simulink model "stm32f0_ccp_sensor"  (Simulink 7.3)
settings: Solver=ode3  SolverMode=SingleTasking  StartTime=0.0  StopTime=10.0  RelTol=1e-3
PreLoadFcn:
  | waijung.modelPreload; % Required for working with Waijung Blockset. Do not remove.
undefined symbols (not defined in the file): ARM, LQFP48, MDK, STM32F072CB
libraries: simulink x216, waijung_soft_i2c_lib x28, waijung_addon_module x12, stm32f0_flash_lib x10, stm32f0_can_lib x3, stm32f0_reset_lib x1, waijung_crc_lib x1, stm32f0_boot_lib x1, stm32f0_device_config_lib x1
(part 1 of 6)
CloseFcn:
  | waijung.modelClose; % Required for working with Waijung Blockset. Do not remove.
settings Model: Creator=Nav  LastModifiedBy=Krisada
settings OptimizationCC: OptimizeModelRefInitCode=on  LifeSpan=1
settings HardwareCC: ProdEndianess=LittleEndian  ProdHWDeviceType=ARM Compatible->Cortex - M0  TargetEndianess=LittleEndian  TargetHWDeviceType=ARM Compatible->Cortex - M0
settings RTWCC: SystemTargetFile=stm32f0.tlc  GenerateMakefile=off  TemplateMakefile=ert_default_tmf  Description=STM32F0 Target  ProcessScript=stm32f0_make_rtw_hook
settings CodeAppCC: IgnoreCustomStorageClasses=off
settings STFCustomTargetCC: ModelReferenceCompliant=off  CombineOutputUpdateFcns=on  ERTCustomFileBanners=on  SupportNonInlinedSFcns=off  SystemTargetFile=stm32f0.tlc
settings ERTTargetCC: MultiwordLength=2048  ModelReferenceCompliant=off  ParMdlRefBuildCompliant=off  CompOptLevelCompliant=off  ERTFirstTimeCompliant=off  SupportContinuousTime=on  ModelStepFunctionPrototypeControlCompliant=off  CPPClassGenCompliant=off  ExtModeMexFile=noextcomm  InlinedParameterPlacement=NonHierarchical  ERTSrcFileBannerTemplate=stm32f0_code_template.cgt  ERTHdrFileBannerTemplate=stm32f0_code_template.cgt  ERTDataSrcFileTemplate=stm32f0_code_template.cgt  ERTDataHdrFileTemplate=stm32f0_code_template.cgt  ERTCustomFileTemplate=stm32f0_file_process.tlc

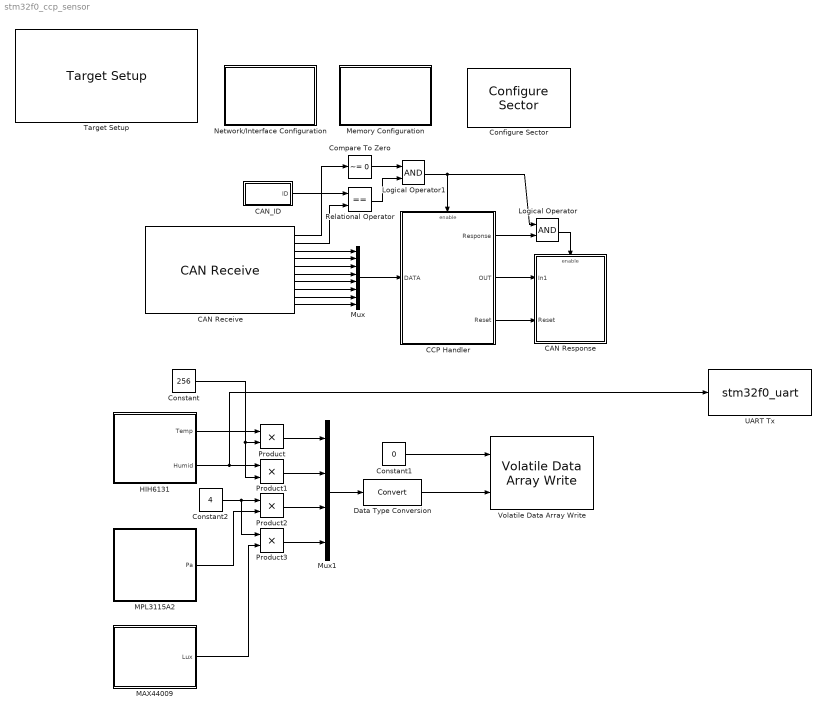
== system stm32f0_ccp_sensor ==
  CAN Receive : stm32f0_can_lib/CAN Receive  conf=Rx  canmodule=1  idtype=Standard  filtertype=Mask  id=0  idmask=0  enableisr=off  usedlc=off  datatype=single  data0type=uint8  data1type=uint8  data2type=uint8  data3type=uint8  data4type=uint8  data5type=uint8  data6type=uint8  data7type=uint8  buffersize=8  sampletime=0.01  sampletimestr=0.01  blockid=CANReceive  inputarray=[]  inputlabelarray={}  outputarray=[ 5, 7, 3, 3, 3, 3, 3, 3, 3, 3]  outputlabelarray={ 'Msg Pending','ID', 'D0 (uint8)', 'D1 (uint8)', 'D2 (uint8)', 'D3 (uint8)', 'D4 (uint8)', 'D5 (uint8)', 'D6 (uint8)', 'D7 (uint8)' }  compat=0  confstr="[\"Standard\",\"Mask\",\"0\",\"0\",\"off\",\"uint8\",\"uint8\",\"uint8\",\"uint8\",\"uint8\",\"uint8\",\"uint8\",\"uint8\",\"8\",\"0\",\"0\",\"0\",\"4\"]"
  CAN Response : Subsystem
  CAN_ID : Subsystem
  CCP Handler : Subsystem  TreatAsAtomicUnit=on
  Compare To Zero : simulink/Logic and Bit Operations/Compare To Zero  SystemSampleTime=-1  relop=~=  LogicOutDataTypeMode=uint8  ZeroCross=off
  Configure Sector : stm32f0_boot_lib/Configure Sector  conf=Configure  flashorigin=0x8004000  flashlength=0x00D000  enableisr=off  usersector=Sector 5: 0x08020000 - 0x0803FFFF  sampletime=-1  sampletimestr=0.01  blockid=ConfigureSector  inputarray=[]  inputlabelarray={}  outputarray=[]  outputlabelarray={}  compat=0  confstr="[\"8020000\",\"5\",\"8004000\"]"
  Constant : Constant  Value=256  OutDataTypeMode=uint32  OutDataType=fixdt(1, 16)  OutScaling=2^0  OutDataTypeStr=uint32
  Constant1 : Constant  Value=0  OutDataTypeMode=uint32  OutDataType=fixdt(1, 16)  OutScaling=2^0  OutDataTypeStr=uint32
  Constant2 : Constant  Value=4  OutDataTypeMode=uint32  OutDataType=fixdt(1, 16)  OutScaling=2^0  OutDataTypeStr=uint32
  Data Type Conversion : DataTypeConversion  OutDataType=fixdt(1, 16)  OutScaling=2^0
  HIH6131 : Subsystem
  Logical Operator : Logic  AllPortsSameDT=off  OutDataTypeMode=boolean  LogicDataType=fixdt(0, 8)  OutDataTypeStr=boolean
  Logical Operator1 : Logic  AllPortsSameDT=off  OutDataTypeMode=boolean  LogicDataType=fixdt(0, 8)  OutDataTypeStr=boolean
  MAX44009 : Subsystem
  MPL3115A2 : Subsystem
  Memory Configuration : Subsystem
  Mux : Mux  Inputs=8
  Mux1 : Mux
  Network/Interface Configuration : Subsystem
  Product{,1..3} (4 alike) : Product  OutDataType=fixdt(1, 16)  OutScaling=2^0  RndMeth=Zero
  Relational Operator : RelationalOperator  Operator===  LogicOutDataTypeMode=boolean  LogicDataType=fixdt(0, 8)  OutDataTypeStr=boolean
  Target Setup : stm32f0_device_config_lib/Target Setup  Priority=100  compiler=MDK-ARM  previous_compiler=MDK-ARM  mcu=STM32F072CB (LQFP48)  mcustr=STM32F072CB  stdlib=STM32F072  clockconfig=STM32F072B-DISCO Default (HSIOSC-8MHz/HCLK-48MHz)  system_stm32f0xx_c_path=F:\trunk\targets\stm32f0_target\stm32f0\utils\STM32F0xx_AN4055\stm32f0_default\hsi8mhz_pll_hclk48mhz  showmemoryconfiguration=on  stacksize=0x400  heapsize=0x200  enableautocompiledownload=on  fullchiperase=off  programmerinterface=None  editctrlstr=on  compilercontrolstr=-c --cpu Cortex-M0 -O3 --apcs=interwork --split_sections $(INCLUDES)  assemblercontrolstr=--cpu Cortex-M0 --apcs=interwork --xref $(INCLUDES)  linkercontrolstr="--cpu Cortex-M0 --strict --scatter \"$(MODELNAME).sct\" --summary_stderr --info summarysizes --map --xref --callgraph --symbols --info sizes --info totals --info unused --info veneers  --list \".\\$(MODELNAME).map\" -o $(MODELNAME).axf"  runafterdownload=on  execprofile=None  profileruart=3  profilerbaud=500000  profilertxpin=Not used  profilerinitstr=0.01,48000000,480000,500000,0  manualsetsampletime=on  sampletime=0.01  blockid=TargetSetup  systickreloadvalue=480000  hseval=8000000  lastprofileruart=3  hclk=48000000  flashorigin=0x8004000  flashlength=0x00D000  ramorigin=0x20000000  ramlength=0x00004000  useextram=off
  UART Tx : S-Function  FunctionName=stm32f0_uart  Parameters=conf,inputporttype,inputportwidth,outputporttype,outputportwidth,asciiheader,optionstring,headerstring,terminatorstring,asciidatatypestring,sampletime,blockid  EnableBusSupport=off  mask(stm32f0_uart){conf=Tx, uartmodule=1, baudrate=115200, databits=8, parity=No, stopbit=1, remaptxpin=A9, remaprxpin=A10, flowcontrol=None, remapctspin=Not used, remaprtspin=Not used, advanceoptions=off, rxbuffersize=64, txbuffersize=64, transfer=Non-Blocking, packetmode=Ascii, binheader='7E 7E', binterminator='03 03', porttype_double=0, porttype_single=0, porttype_int8=0, porttype_uint8=0, porttype_int16=0, porttype_uint16=0, porttype_int32=0, porttype_uint32=2, asciiformat='%1.2f', rx_asciiterminator=CR (0x0D - "\r"), tx_asciiterminator=CRLF (0x0D 0x0A - "\r\n"), storagename=<empty>, varname=, asciiheader=%1.2f\r\n, sampletime=inf, enablecustomportlabel=off, cinputportlabel=de, coutputportlabel=fff,ff,sdfsd, portpinstr=0, blockid=UARTTx, inputporttype=[ -1], inputportwidth=[], inputportlabel={ '%f'}, outputporttype=[], outputportwidth=[], outputportlabel={}, compat=0, optionstring=["1", "1", "A", "9", "1", "A", "10", "0", "*", "*", "0", "*", "*", "1", "1", "", "", "115200", "8", "No", "1", "None", "3", "2", "64", "64", "Ascii", "Non-Blocking", ""], headerstring=[], terminatorstring=["13","10"], asciidatatypestring=["float"], lastmodule=1}
      mask prompts: conf "Configuration"; uartmodule "UART Module"; baudrate "Baud rate (bps)"; databits "Data bits"; stopbit "Stop bit"; remaptxpin "Tx pin"; remaprxpin "Rx pin"; flowcontrol "Hardware flow control"; remapctspin "HW Flow control, CTS Pin"; remaprtspin "HW Flow control, RTS Pin"; advanceoptions "Advance options"; rxbuffersize "Rx buffer size (bytes)"; txbuffersize "Tx buffer size (bytes)"; packetmode "Packet mode"; binheader "Binary header (example: '7E 7E')"; binterminator "Binary terminator (example: '03 03')"; porttype_double "Number of data port, type DOUBLE"; porttype_single "Number of data port, type SINGLE"; porttype_int8 "Number of data port, type INT8"; porttype_uint8 "Number of data port, type UINT8"; porttype_int16 "Number of data port, type INT16"; porttype_uint16 "Number of data port, type UINT16"; porttype_int32 "Number of data port, type INT32"; porttype_uint32 "Number of data port, type UINT32"; asciiformat "Ascii format"; rx_asciiterminator "End of packet"; tx_asciiterminator "End of packet"; storagename "Buffer"; varname "Var name"; asciiheader "Ascii header (printf format)"; sampletime "Sample time (sec)"; enablecustomportlabel "Enable custom port labels (Ex. In1, In2, In3)"; cinputportlabel "Custom input port labels (Ex. In1, In2, In3)"; coutputportlabel "Custom output port labels (Ex. Out1, Out2, Out3)"; portpinstr "Port Pin String"; blockid "Block ID"; inputporttype "Input Port Type"; inputportwidth "Input Port Width"; inputportlabel "Input Port Label"; outputporttype "Output Port Type"; outputportwidth "Output Port Width"; outputportlabel "Output port label"; compat "Compatibility (Reserved for future use)"; optionstring "String(s) to be passed to TLC"; lastmodule "Last module selected"
      mask help:
      | UART Module
      |  - Select module corresponding to "UART Setup" block.
      | Transfer
      |  - Blocking: after write DMA buffer, the block wait until buffer empty.
      |  - Non-Blocking: the block will not wait for buffer empty.
      | Packet mode:
      |  - Ascii: sending data is ascii, Ascii format + End of packet.
      |  - Binary: sending data is binary format, Header + Data + Terminator
      |  - String Buffer: Volatile Data Storage variable name as sending data.
      | Ascii format:
      |  - %U, %I, %D, %O, %X, %u, %i, %d, %o, %x: Uint32
      |  - %E, %G, %F, %e, %g, %f: Single
      |  - %C, %c: Int8
      |  - %S, %s: (char *), this port is output of Volatile Data Storage Read block, which data type is string.
      mask init:
      | stm32f0_uart_callback('init');
      mask Help: web(fullfile(waijungdocroot,'stm32f0_uart_tx.htm'), '-browser')
      mask StyleString: popup(Setup|Tx|Rx),popup(1|2|3|4),edit,popup(8),popup(No|Odd|Even),popup(0.5|1|1.5|2),popup(Not used|A9|B6),popup(Not used|A10|B7),popup(None|RTS|CTS|RTS/CTS),popup(Not used|A11),popup(Not used|A12),checkbox,popup(16|32|64|128|256|512),popup(16|32|64|128|256|512),popup(Blocking|Non-Blocking),popup(Ascii|Binary|String Buffer),edit,edit,edit,edit,edit,edit,edit,edit,edit,edit,edit,popup(CR (0x0D - "\r")|LF (0x0A - "\n")|CRLF (0x0D 0x0A - "\r\n")),popup(CR (0x0D - "\r")|LF (0x0A - "\n")|CRLF (0x0D 0x0A - "\r\n")|None),popup(<empty>),edit,edit,edit,checkbox,edit,edit,edit,edit,edit,edit,edit,edit,edit,edit,edit,edit,edit,edit,edit,edit
      mask CallbackString: stm32f0_uart_callback('conf');|stm32f0_uart_callback('uartmodule');|||||||stm32f0_uart_callback('flowcontrol');|||stm32f0_uart_callback('advanceoptions');|||stm32f0_uart_callback('conf');|stm32f0_uart_callback('conf');|stm32f0_uart_callback('binheader');|stm32f0_uart_callback('binterminator');|||||||||stm32f0_uart_callback('asciiformat');|||stm32f0_uart_callback('storagename');|||stm32f0_uart_callback('sampletime');|stm32f0_uart_callback('enablecustomportlabel');|stm32f0_uart_callback('conf');|stm32f0_uart_callback('conf');||stm32f0_uart_callback('blockid');||||||||||||
      mask Display: text(0.95, 0.5, 'Module: USART1_Tx\nPacket: Ascii\nTransfer: Non-Blocking\nTs (sec): 0.5','ver','middle','hor','right'); port_label('input', 1,'%f');
  Volatile Data Array Write : waijung_addon_module/Data Storage/Volatile Data Array Write  conf=Write  specificaddress=off  storagename=READ_DATA  memoryaddress=hex2dec('64000000')  storagetype=uint8  datasize=120*160*3  varname=VolatileDataArray_READ_DATA  datatype=uint32  datacount=4  variablesize=off  portpinstr=0  sampletime=inf  blockid=VolatileDataArrayWrite  inputporttype=[7 7]  inputportwidth=[1 4]  inputportlabel={'Offset', 'Data'}  outputporttype=[]  outputportwidth=[]  outputportlabel={}  compat=0  optionstring="[\"READ_DATA\",\"uint8\",\"256\",\"VolatileDataArray_READ_DATA\",\"uint8_t\",\"uint32\",\"uint32_t\",\"4\",\"Param1\"]"
  wires:
  CAN Receive/1 -> Compare To Zero/1
  CAN Receive/3 -> Mux/1
  CAN Receive/4 -> Mux/2
  CAN Receive/5 -> Mux/3
  CAN Receive/6 -> Mux/4
  CAN Receive/7 -> Mux/5
  CAN Receive/8 -> Mux/6
  CAN Receive/9 -> Mux/7
  CAN Receive/10 -> Mux/8
  Mux/1 -> CCP Handler/1(DATA)
  CAN Receive/2 -> Relational Operator/2
  CCP Handler/2(OUT) -> CAN Response/1(In1)
  CCP Handler/1(Response) -> Logical Operator/2
  Logical Operator/1 -> CAN Response/Enable
  CCP Handler/3(Reset) -> CAN Response/2(Reset)
  CAN_ID/1(ID) -> Relational Operator/1
  Compare To Zero/1 -> Logical Operator1/1
  Logical Operator1/1 -> CCP Handler/Enable, Logical Operator/1
  Mux1/1 -> Data Type Conversion/1
  Product/1 -> Mux1/1
  Product1/1 -> Mux1/2
  Constant/1 -> Product/2, Product1/2
  Relational Operator/1 -> Logical Operator1/2
  HIH6131/1(Temp) -> Product/1
  HIH6131/2(Humid) -> Product1/1, UART Tx/1
  Product2/1 -> Mux1/3
  Constant2/1 -> Product2/1, Product3/1
  MPL3115A2/1(Pa) -> Product2/2
  Product3/1 -> Mux1/4
  MAX44009/1(Lux) -> Product3/2
  Constant1/1 -> Volatile Data Array Write/1
  Data Type Conversion/1 -> Volatile Data Array Write/2

== system stm32f0_ccp_sensor/CAN Response ==
  In1 : Inport
  Reset : Inport  Port=2
  Enable : EnablePort
  CAN Transmit : stm32f0_can_lib/CAN Transmit  conf=Tx  canmodule=1  transfer=Blocking  timeout=0.1  idtype=Standard  specificid=on  id=255  specificdlc=on  dlc=8  enablestatus=on  datatype=single  data0type=uint8  data1type=uint8  data2type=uint8  data3type=uint8  data4type=uint8  data5type=uint8  data6type=uint8  data7type=uint8  inputarray=[ 3, 3, 3, 3, 3, 3, 3, 3]  inputlabelarray={ 'D0 (uint8)', 'D1 (uint8)', 'D2 (uint8)', 'D3 (uint8)', 'D4 (uint8)', 'D5 (uint8)', 'D6 (uint8)', 'D7 (uint8)' }  outputarray=[7]  outputlabelarray={'Status'}  sampletime=-1  sampletimestr=0.01  blockid=CANResponseCANTransmit  compat=0  confstr="[\"Blocking\",\"0.1\",\"Standard\",\"on\",\"255\",\"on\",\"8\",\"on\",\"uint8\",\"uint8\",\"uint8\",\"uint8\",\"uint8\",\"uint8\",\"uint8\",\"uint8\"]"
  Compare To Zero : simulink/Logic and Bit Operations/Compare To Zero  SystemSampleTime=-1  relop===  LogicOutDataTypeMode=boolean  ZeroCross=off
  Demux : Demux  Outputs=8
  Demux1 : Demux  Outputs=8
  Logical Operator : Logic  AllPortsSameDT=off  OutDataTypeMode=boolean  LogicDataType=fixdt(0, 8)  OutDataTypeStr=boolean
  Reboot : Subsystem  TreatAsAtomicUnit=on
  UART Tx : S-Function  FunctionName=stm32f0_uart  Parameters=conf,inputporttype,inputportwidth,outputporttype,outputportwidth,asciiheader,optionstring,headerstring,terminatorstring,asciidatatypestring,sampletime,blockid  EnableBusSupport=off  mask(stm32f0_uart){conf=Tx, uartmodule=1, baudrate=115200, databits=8, parity=No, stopbit=1, remaptxpin=A9, remaprxpin=A10, flowcontrol=None, remapctspin=Not used, remaprtspin=Not used, advanceoptions=off, rxbuffersize=64, txbuffersize=64, transfer=Non-Blocking, packetmode=Ascii, binheader='7E 7E', binterminator='03 03', porttype_double=0, porttype_single=0, porttype_int8=0, porttype_uint8=0, porttype_int16=0, porttype_uint16=0, porttype_int32=0, porttype_uint32=2, asciiformat='TX: %X,%X,%X,%X,%X,%X,%X,%X: %u', rx_asciiterminator=CR (0x0D - "\r"), tx_asciiterminator=CRLF (0x0D 0x0A - "\r\n"), storagename=<empty>, varname=, asciiheader=TX: %X,%X,%X,%X,%X,%X,%X,%X: %u\r\n, sampletime=inf, enablecustomportlabel=off, cinputportlabel=de, coutputportlabel=fff,ff,sdfsd, portpinstr=0, blockid=CANResponseUARTTx, inputporttype=[ -1 -1 -1 -1 -1 -1 -1 -1 -1], inputportwidth=[], inputportlabel={ '%X' '%X' '%X' '%X' '%X' '%X' '%X' '%X' '%u'}, outputporttype=[], outputportwidth=[], outputportlabel={}, compat=0, optionstring=["1", "1", "A", "9", "1", "A", "10", "0", "*", "*", "0", "*", "*", "1", "1", "", "", "115200", "8", "No", "1", "None", "3", "2", "64", "64", "Ascii", "Non-Blocking", ""], headerstring=[], terminatorstring=["13","10"], asciidatatypestring=["uint32_t","uint32_t","uint32_t","uint32_t","uint32_t","uint32_t","uint32_t","uint32_t","uint32_t"], lastmodule=1}
      mask prompts: conf "Configuration"; uartmodule "UART Module"; baudrate "Baud rate (bps)"; databits "Data bits"; stopbit "Stop bit"; remaptxpin "Tx pin"; remaprxpin "Rx pin"; flowcontrol "Hardware flow control"; remapctspin "HW Flow control, CTS Pin"; remaprtspin "HW Flow control, RTS Pin"; advanceoptions "Advance options"; rxbuffersize "Rx buffer size (bytes)"; txbuffersize "Tx buffer size (bytes)"; packetmode "Packet mode"; binheader "Binary header (example: '7E 7E')"; binterminator "Binary terminator (example: '03 03')"; porttype_double "Number of data port, type DOUBLE"; porttype_single "Number of data port, type SINGLE"; porttype_int8 "Number of data port, type INT8"; porttype_uint8 "Number of data port, type UINT8"; porttype_int16 "Number of data port, type INT16"; porttype_uint16 "Number of data port, type UINT16"; porttype_int32 "Number of data port, type INT32"; porttype_uint32 "Number of data port, type UINT32"; asciiformat "Ascii format"; rx_asciiterminator "End of packet"; tx_asciiterminator "End of packet"; storagename "Buffer"; varname "Var name"; asciiheader "Ascii header (printf format)"; sampletime "Sample time (sec)"; enablecustomportlabel "Enable custom port labels (Ex. In1, In2, In3)"; cinputportlabel "Custom input port labels (Ex. In1, In2, In3)"; coutputportlabel "Custom output port labels (Ex. Out1, Out2, Out3)"; portpinstr "Port Pin String"; blockid "Block ID"; inputporttype "Input Port Type"; inputportwidth "Input Port Width"; inputportlabel "Input Port Label"; outputporttype "Output Port Type"; outputportwidth "Output Port Width"; outputportlabel "Output port label"; compat "Compatibility (Reserved for future use)"; optionstring "String(s) to be passed to TLC"; lastmodule "Last module selected"
      mask help:
      | UART Module
      |  - Select module corresponding to "UART Setup" block.
      | Transfer
      |  - Blocking: after write DMA buffer, the block wait until buffer empty.
      |  - Non-Blocking: the block will not wait for buffer empty.
      | Packet mode:
      |  - Ascii: sending data is ascii, Ascii format + End of packet.
      |  - Binary: sending data is binary format, Header + Data + Terminator
      |  - String Buffer: Volatile Data Storage variable name as sending data.
      | Ascii format:
      |  - %U, %I, %D, %O, %X, %u, %i, %d, %o, %x: Uint32
      |  - %E, %G, %F, %e, %g, %f: Single
      |  - %C, %c: Int8
      |  - %S, %s: (char *), this port is output of Volatile Data Storage Read block, which data type is string.
      mask init:
      | stm32f0_uart_callback('init');
      mask Help: web(fullfile(waijungdocroot,'stm32f0_uart_tx.htm'), '-browser')
      mask StyleString: popup(Setup|Tx|Rx),popup(1|2|3|4),edit,popup(8),popup(No|Odd|Even),popup(0.5|1|1.5|2),popup(Not used|A9|B6),popup(Not used|A10|B7),popup(None|RTS|CTS|RTS/CTS),popup(Not used|A11),popup(Not used|A12),checkbox,popup(16|32|64|128|256|512),popup(16|32|64|128|256|512),popup(Blocking|Non-Blocking),popup(Ascii|Binary|String Buffer),edit,edit,edit,edit,edit,edit,edit,edit,edit,edit,edit,popup(CR (0x0D - "\r")|LF (0x0A - "\n")|CRLF (0x0D 0x0A - "\r\n")),popup(CR (0x0D - "\r")|LF (0x0A - "\n")|CRLF (0x0D 0x0A - "\r\n")|None),popup(<empty>),edit,edit,edit,checkbox,edit,edit,edit,edit,edit,edit,edit,edit,edit,edit,edit,edit,edit,edit,edit,edit
      mask CallbackString: stm32f0_uart_callback('conf');|stm32f0_uart_callback('uartmodule');|||||||stm32f0_uart_callback('flowcontrol');|||stm32f0_uart_callback('advanceoptions');|||stm32f0_uart_callback('conf');|stm32f0_uart_callback('conf');|stm32f0_uart_callback('binheader');|stm32f0_uart_callback('binterminator');|||||||||stm32f0_uart_callback('asciiformat');|||stm32f0_uart_callback('storagename');|||stm32f0_uart_callback('sampletime');|stm32f0_uart_callback('enablecustomportlabel');|stm32f0_uart_callback('conf');|stm32f0_uart_callback('conf');||stm32f0_uart_callback('blockid');||||||||||||
      mask Display: text(0.95, 0.5, 'Module: USART1_Tx\nPacket: Ascii\nTransfer: Non-Blocking\nTs (sec): 0.01','ver','middle','hor','right'); port_label('input', 1,'%X'); port_label('input', 2,'%X'); port_label('input', 3,'%X'); port_label('input', 4,'%X'); port_label('input', 5,'%X'); port_label('input', 6,'%X'); port_label('input', 7,'%X'); port_label('input', 8,'%X'); port_label('input', 9,'%u');
  wires:
  Demux/1 -> CAN Transmit/1
  Demux/2 -> CAN Transmit/2
  Demux/3 -> CAN Transmit/3
  Demux/4 -> CAN Transmit/4
  Demux/5 -> CAN Transmit/5
  Demux/6 -> CAN Transmit/6
  Demux/7 -> CAN Transmit/7
  Demux/8 -> CAN Transmit/8
  In1/1 -> Demux/1, Demux1/1
  CAN Transmit/1 -> Compare To Zero/1
  Compare To Zero/1 -> Logical Operator/1, UART Tx/9
  Reset/1 -> Logical Operator/2
  Logical Operator/1 -> Reboot/Enable
  Demux1/1 -> UART Tx/1
  Demux1/2 -> UART Tx/2
  Demux1/3 -> UART Tx/3
  Demux1/4 -> UART Tx/4
  Demux1/5 -> UART Tx/5
  Demux1/6 -> UART Tx/6
  Demux1/7 -> UART Tx/7
  Demux1/8 -> UART Tx/8

== system stm32f0_ccp_sensor/CAN_ID ==
  Memory : Memory  X0=1  InheritSampleTime=on  LinearizeMemory=on
  Subsystem : Subsystem
  ID : Outport
  wires:
  Subsystem/2(ID) -> ID/1
  Memory/1 -> Subsystem/Enable
  Subsystem/1(FirstTime) -> Memory/1

== system stm32f0_ccp_sensor/CCP Handler ==
  DATA : Inport  OutDataType=fixdt(1, 16)  OutScaling=2^0
  Enable : EnablePort
  CRO CONNECT Parser : Subsystem
  CRO MTA Parser : Subsystem
  CRO UNLOCK Parser : Subsystem
  Command Processing : Subsystem  TreatAsAtomicUnit=on
  Constant : Constant  Value=0  OutDataTypeMode=uint8  OutDataType=fixdt(1, 16)  OutScaling=2^0  OutDataTypeStr=uint8
  Demux : Demux  Outputs=8
  Mux : Mux  Inputs=3
  Mux1 : Mux
  Switch : Switch  Criteria=u2 ~= 0  OutDataType=fixdt(1, 16)  OutScaling=2^0
  UART Tx : S-Function  FunctionName=stm32f0_uart  Parameters=conf,inputporttype,inputportwidth,outputporttype,outputportwidth,asciiheader,optionstring,headerstring,terminatorstring,asciidatatypestring,sampletime,blockid  EnableBusSupport=off  mask(stm32f0_uart){conf=Tx, uartmodule=1, baudrate=115200, databits=8, parity=No, stopbit=1, remaptxpin=A9, remaprxpin=A10, flowcontrol=None, remapctspin=Not used, remaprtspin=Not used, advanceoptions=off, rxbuffersize=64, txbuffersize=64, transfer=Non-Blocking, packetmode=Ascii, binheader='7E 7E', binterminator='03 03', porttype_double=0, porttype_single=0, porttype_int8=0, porttype_uint8=0, porttype_int16=0, porttype_uint16=0, porttype_int32=0, porttype_uint32=2, asciiformat='RX: %X,%X,%X,%X,%X,%X,%X,%X', rx_asciiterminator=CR (0x0D - "\r"), tx_asciiterminator=CRLF (0x0D 0x0A - "\r\n"), storagename=<empty>, varname=, asciiheader=RX: %X,%X,%X,%X,%X,%X,%X,%X\r\n, sampletime=inf, enablecustomportlabel=off, cinputportlabel=de, coutputportlabel=fff,ff,sdfsd, portpinstr=0, blockid=CCPHandlerUARTTx, inputporttype=[ -1 -1 -1 -1 -1 -1 -1 -1], inputportwidth=[], inputportlabel={ '%X' '%X' '%X' '%X' '%X' '%X' '%X' '%X'}, outputporttype=[], outputportwidth=[], outputportlabel={}, compat=0, optionstring=["1", "1", "A", "9", "1", "A", "10", "0", "*", "*", "0", "*", "*", "1", "1", "", "", "115200", "8", "No", "1", "None", "3", "2", "64", "64", "Ascii", "Non-Blocking", ""], headerstring=[], terminatorstring=["13","10"], asciidatatypestring=["uint32_t","uint32_t","uint32_t","uint32_t","uint32_t","uint32_t","uint32_t","uint32_t"], lastmodule=1}
      mask prompts: conf "Configuration"; uartmodule "UART Module"; baudrate "Baud rate (bps)"; databits "Data bits"; stopbit "Stop bit"; remaptxpin "Tx pin"; remaprxpin "Rx pin"; flowcontrol "Hardware flow control"; remapctspin "HW Flow control, CTS Pin"; remaprtspin "HW Flow control, RTS Pin"; advanceoptions "Advance options"; rxbuffersize "Rx buffer size (bytes)"; txbuffersize "Tx buffer size (bytes)"; packetmode "Packet mode"; binheader "Binary header (example: '7E 7E')"; binterminator "Binary terminator (example: '03 03')"; porttype_double "Number of data port, type DOUBLE"; porttype_single "Number of data port, type SINGLE"; porttype_int8 "Number of data port, type INT8"; porttype_uint8 "Number of data port, type UINT8"; porttype_int16 "Number of data port, type INT16"; porttype_uint16 "Number of data port, type UINT16"; porttype_int32 "Number of data port, type INT32"; porttype_uint32 "Number of data port, type UINT32"; asciiformat "Ascii format"; rx_asciiterminator "End of packet"; tx_asciiterminator "End of packet"; storagename "Buffer"; varname "Var name"; asciiheader "Ascii header (printf format)"; sampletime "Sample time (sec)"; enablecustomportlabel "Enable custom port labels (Ex. In1, In2, In3)"; cinputportlabel "Custom input port labels (Ex. In1, In2, In3)"; coutputportlabel "Custom output port labels (Ex. Out1, Out2, Out3)"; portpinstr "Port Pin String"; blockid "Block ID"; inputporttype "Input Port Type"; inputportwidth "Input Port Width"; inputportlabel "Input Port Label"; outputporttype "Output Port Type"; outputportwidth "Output Port Width"; outputportlabel "Output port label"; compat "Compatibility (Reserved for future use)"; optionstring "String(s) to be passed to TLC"; lastmodule "Last module selected"
      mask help:
      | UART Module
      |  - Select module corresponding to "UART Setup" block.
      | Transfer
      |  - Blocking: after write DMA buffer, the block wait until buffer empty.
      |  - Non-Blocking: the block will not wait for buffer empty.
      | Packet mode:
      |  - Ascii: sending data is ascii, Ascii format + End of packet.
      |  - Binary: sending data is binary format, Header + Data + Terminator
      |  - String Buffer: Volatile Data Storage variable name as sending data.
      | Ascii format:
      |  - %U, %I, %D, %O, %X, %u, %i, %d, %o, %x: Uint32
      |  - %E, %G, %F, %e, %g, %f: Single
      |  - %C, %c: Int8
      |  - %S, %s: (char *), this port is output of Volatile Data Storage Read block, which data type is string.
      mask init:
      | stm32f0_uart_callback('init');
      mask Help: web(fullfile(waijungdocroot,'stm32f0_uart_tx.htm'), '-browser')
      mask StyleString: popup(Setup|Tx|Rx),popup(1|2|3|4),edit,popup(8),popup(No|Odd|Even),popup(0.5|1|1.5|2),popup(Not used|A9|B6),popup(Not used|A10|B7),popup(None|RTS|CTS|RTS/CTS),popup(Not used|A11),popup(Not used|A12),checkbox,popup(16|32|64|128|256|512),popup(16|32|64|128|256|512),popup(Blocking|Non-Blocking),popup(Ascii|Binary|String Buffer),edit,edit,edit,edit,edit,edit,edit,edit,edit,edit,edit,popup(CR (0x0D - "\r")|LF (0x0A - "\n")|CRLF (0x0D 0x0A - "\r\n")),popup(CR (0x0D - "\r")|LF (0x0A - "\n")|CRLF (0x0D 0x0A - "\r\n")|None),popup(<empty>),edit,edit,edit,checkbox,edit,edit,edit,edit,edit,edit,edit,edit,edit,edit,edit,edit,edit,edit,edit,edit
      mask CallbackString: stm32f0_uart_callback('conf');|stm32f0_uart_callback('uartmodule');|||||||stm32f0_uart_callback('flowcontrol');|||stm32f0_uart_callback('advanceoptions');|||stm32f0_uart_callback('conf');|stm32f0_uart_callback('conf');|stm32f0_uart_callback('binheader');|stm32f0_uart_callback('binterminator');|||||||||stm32f0_uart_callback('asciiformat');|||stm32f0_uart_callback('storagename');|||stm32f0_uart_callback('sampletime');|stm32f0_uart_callback('enablecustomportlabel');|stm32f0_uart_callback('conf');|stm32f0_uart_callback('conf');||stm32f0_uart_callback('blockid');||||||||||||
      mask Display: text(0.95, 0.5, 'Module: USART1_Tx\nPacket: Ascii\nTransfer: Non-Blocking\nTs (sec): 0.01','ver','middle','hor','right'); port_label('input', 1,'%X'); port_label('input', 2,'%X'); port_label('input', 3,'%X'); port_label('input', 4,'%X'); port_label('input', 5,'%X'); port_label('input', 6,'%X'); port_label('input', 7,'%X'); port_label('input', 8,'%X');
  Response : Outport  OutDataType=fixdt(1, 16)  OutScaling=2^0
  OUT : Outport  Port=2  OutDataType=fixdt(1, 16)  OutScaling=2^0
  Reset : Outport  Port=3  OutDataType=fixdt(1, 16)  OutScaling=2^0
  wires:
  DATA/1 -> CRO CONNECT Parser/1(Data(8)), Demux/1
  CRO CONNECT Parser/2(CMD) -> CRO UNLOCK Parser/2(CMD), CRO MTA Parser/2(CMD), Command Processing/1(CMD)
  CRO CONNECT Parser/3(Data(6)) -> CRO MTA Parser/3(Data(6)), CRO UNLOCK Parser/3(Data(6)), Command Processing/3(Data(6))
  CRO CONNECT Parser/1(Connected) -> CRO MTA Parser/1(Connect), CRO UNLOCK Parser/1(Connect), Switch/2, Command Processing/Enable
  Switch/1 -> Response/1
  Constant/1 -> Switch/3
  Command Processing/2(CAN Tx Data) -> OUT/1
  CRO CONNECT Parser/4(CTR) -> Command Processing/2(CTR)
  Command Processing/1(Response) -> Switch/1
  CRO UNLOCK Parser/1(CAL Unlocked) -> Mux/1
  CRO UNLOCK Parser/2(PGM Unlocked) -> Mux/2
  CRO UNLOCK Parser/3(DAQ Unlocked) -> Mux/3
  Mux1/1 -> Command Processing/4(MTA_Info)
  Mux/1 -> Command Processing/5(Unlock status)
  CRO MTA Parser/1(ValidAddr) -> Mux1/1
  CRO MTA Parser/2(ExtAddr) -> Mux1/2
  CRO MTA Parser/3(MTA) -> Mux1/3
  CRO MTA Parser/4(PostInc_MTA) -> Mux1/4
  Command Processing/3(Reset) -> Reset/1
  Demux/1 -> UART Tx/1
  Demux/2 -> UART Tx/2
  Demux/3 -> UART Tx/3
  Demux/4 -> UART Tx/4
  Demux/5 -> UART Tx/5
  Demux/6 -> UART Tx/6
  Demux/7 -> UART Tx/7
  Demux/8 -> UART Tx/8

== system stm32f0_ccp_sensor/HIH6131 ==
  Bitwise Operator : simulink/Logic and Bit Operations/Bitwise Operator  logicop=AND  UseBitMask=on  BitMask=1  BitMaskRealWorld=Stored Integer
  Constant : Constant  Value=hex2dec('4E')  OutDataTypeMode=uint8  OutDataType=fixdt(1, 16)  OutScaling=2^0  OutDataTypeStr=uint8  SampleTime=0.5
  Counter Free-Running : simulink/Sources/Counter Free-Running  SystemSampleTime=-1  NumBits=16  tsamp=-1
  Logical Operator : Logic  Operator=NOT  AllPortsSameDT=off  OutDataTypeMode=boolean  LogicDataType=fixdt(0, 8)  OutDataTypeStr=boolean
  Read : Subsystem
  Request : Subsystem
  Temp : Outport
  Humid : Outport  Port=2
  wires:
  Constant/1 -> Read/1(In1), Request/1(In1)
  Counter Free-Running/1 -> Bitwise Operator/1
  Bitwise Operator/1 -> Logical Operator/1, Request/Enable
  Logical Operator/1 -> Read/Enable
  Read/1(Humid) -> Humid/1
  Read/2(Temp) -> Temp/1

== system stm32f0_ccp_sensor/MAX44009 ==
  Compare To Zero : simulink/Logic and Bit Operations/Compare To Zero  SystemSampleTime=-1  relop===  LogicOutDataTypeMode=uint8  ZeroCross=off
  Compare To Zero1 : simulink/Logic and Bit Operations/Compare To Zero  SystemSampleTime=-1  relop===  LogicOutDataTypeMode=uint8  ZeroCross=off
  Compare To Zero2 : simulink/Logic and Bit Operations/Compare To Zero  SystemSampleTime=-1  relop===  LogicOutDataTypeMode=uint8  ZeroCross=off
  Enabled Subsystem : Subsystem  TreatAsAtomicUnit=on
  Logical Operator : Logic  Inputs=3  AllPortsSameDT=off  OutDataTypeMode=boolean  LogicDataType=fixdt(0, 8)  OutDataTypeStr=boolean
  Register : Constant  Value=hex2dec('03')  OutDataTypeMode=uint8  OutDataType=fixdt(1, 16)  OutScaling=2^0  OutDataTypeStr=uint8
  Register1 : Constant  Value=hex2dec('04')  OutDataTypeMode=uint8  OutDataType=fixdt(1, 16)  OutScaling=2^0  OutDataTypeStr=uint8
  Register2 : Constant  Value=hex2dec('02')  OutDataTypeMode=uint8  OutDataType=fixdt(1, 16)  OutScaling=2^0  OutDataTypeStr=uint8
  Slave Address : Constant  Value=hex2dec('94')  OutDataTypeMode=uint8  OutDataType=fixdt(1, 16)  OutScaling=2^0  OutDataTypeStr=uint8  SampleTime=0.5
  Soft I2C Master Read/Write : waijung_soft_i2c_lib/Soft I2C Master Read//Write  conf=ReadWrite  targetname=stm32f0  module=1  transfer=Blocking  clk=100  timeout=25  sdapins={'A4','A6'}  sclpins='A5'  writecount=1  readcount=1  waittime=0  forcestop=off  portpinstr=0  sampletime=inf  blockid=MAX44009SoftI2CMasterReadWrite  inputporttype=[3 3]  inputportwidth=[]  inputportlabel={'SlvAddr' 'Wr0 (uint8)'}  outputporttype=[3 3 ]  outputportwidth=[1 1]  outputportlabel={'Status' 'Rd0 (uint8)'}  compat=0  optionstring="[\"1\",\"1\",\"1\",\"0\",\"off\",\"1\"]"
  Soft I2C Master Read/Write1 : waijung_soft_i2c_lib/Soft I2C Master Read//Write  conf=ReadWrite  targetname=stm32f0  module=1  transfer=Blocking  clk=100  timeout=25  sdapins={'A4','A6'}  sclpins='A5'  writecount=1  readcount=1  waittime=0  forcestop=off  portpinstr=0  sampletime=inf  blockid=MAX44009SoftI2CMasterReadWrite1  inputporttype=[3 3]  inputportwidth=[]  inputportlabel={'SlvAddr' 'Wr0 (uint8)'}  outputporttype=[3 3 ]  outputportwidth=[1 1]  outputportlabel={'Status' 'Rd0 (uint8)'}  compat=0  optionstring="[\"1\",\"1\",\"1\",\"0\",\"off\",\"1\"]"
  Soft I2C Master Read/Write2 : waijung_soft_i2c_lib/Soft I2C Master Read//Write  conf=ReadWrite  targetname=stm32f0  module=1  transfer=Blocking  clk=100  timeout=25  sdapins={'A4','A6'}  sclpins='A5'  writecount=1  readcount=1  waittime=0  forcestop=off  portpinstr=0  sampletime=inf  blockid=MAX44009SoftI2CMasterReadWrite2  inputporttype=[3 3]  inputportwidth=[]  inputportlabel={'SlvAddr' 'Wr0 (uint8)'}  outputporttype=[3 3 ]  outputportwidth=[1 1]  outputportlabel={'Status' 'Rd0 (uint8)'}  compat=0  optionstring="[\"1\",\"1\",\"1\",\"0\",\"off\",\"1\"]"
  Terminator : Terminator
  Lux : Outport  OutDataType=fixdt(1, 16)  OutScaling=2^0
  wires:
  Enabled Subsystem/2(CDR) -> Terminator/1
  Enabled Subsystem/1(Lux) -> Lux/1
  Soft I2C Master Read/Write1/1 -> Compare To Zero/1
  Register/1 -> Soft I2C Master Read/Write1/2
  Slave Address/1 -> Soft I2C Master Read/Write1/1, Soft I2C Master Read/Write2/1, Soft I2C Master Read/Write/1
  Register1/1 -> Soft I2C Master Read/Write2/2
  Soft I2C Master Read/Write2/1 -> Compare To Zero1/1
  Logical Operator/1 -> Enabled Subsystem/Enable
  Soft I2C Master Read/Write1/2 -> Enabled Subsystem/2(MSB)
  Soft I2C Master Read/Write2/2 -> Enabled Subsystem/3(LSB)
  Register2/1 -> Soft I2C Master Read/Write/2
  Soft I2C Master Read/Write/1 -> Compare To Zero2/1
  Compare To Zero/1 -> Logical Operator/2
  Compare To Zero2/1 -> Logical Operator/1
  Compare To Zero1/1 -> Logical Operator/3
  Soft I2C Master Read/Write/2 -> Enabled Subsystem/1(Configuration)

== system stm32f0_ccp_sensor/MPL3115A2 ==
  Constant : Constant  Value=hex2dec('C0')  OutDataTypeMode=uint8  OutDataType=fixdt(1, 16)  OutScaling=2^0  OutDataTypeStr=uint8  SampleTime=0.5
  Convert : Subsystem
  MPL3115A2_Initialize : Subsystem
  Reading : Subsystem  TreatAsAtomicUnit=on
  Terminator : Terminator
  Terminator1 : Terminator
  Pa : Outport
  wires:
  Constant/1 -> MPL3115A2_Initialize/1(SlvAddr), Reading/1(SlvAddr)
  Reading/1(DATA_VALID) -> Convert/Enable
  Reading/6(T_LSB) -> Terminator1/1
  Reading/5(T_MSB) -> Terminator/1
  Reading/4(P_LSB) -> Convert/3(In3)
  Reading/3(P_CSB) -> Convert/2(In2)
  Reading/2(P_MSB) -> Convert/1(In1)
  MPL3115A2_Initialize/1(SETUP_READY) -> Reading/Enable
  Convert/1(Pa) -> Pa/1

== system stm32f0_ccp_sensor/Memory Configuration ==
  EEP Emulation Storage : S-Function  FunctionName=stm32f0_eep_emulation  Parameters=conf,inputporttype,inputportwidth,outputporttype,outputportwidth,eepfilename,eepinfo,varname,optionstring,sampletime,blockid  EnableBusSupport=off  mask(stm32f0_eep_emulation){conf=Setup, datatype=uint32, storagedefinename='CAN_ID', storagename=<empty>, varname='<empty>', initialvalue=[0], storageindex=-1, eepfilename='stm32f0_ccp_sensor.eeprom', eepinfo='', sampletime=inf, enablecustomportlabel=off, cinputportlabel=0, coutputportlabel=, portpinstr=0, blockid=MemoryConfigurationEEPEmulationStorage, inputporttype=[], inputportwidth=[], inputportlabel={}, outputporttype=[], outputportwidth=[], outputportlabel={}, compat=0, optionstring=[]}
      mask prompts: conf "Configuration"; datatype "Storage type"; storagedefinename "Storage name"; storagename "Storage name"; varname "Var name (hidden)"; initialvalue "Initial value"; storageindex "Storage name index (hidden)"; eepfilename "EEP file name (hidden)"; eepinfo "EEP Information (hidden), [name, initialvalue, datatype]"; sampletime "Sample time (sec)"; enablecustomportlabel "Enable custom port labels (Ex. In1, In2, In3)"; cinputportlabel "Custom input port labels (Ex. In1, In2, In3)"; coutputportlabel "Custom output port labels (Ex. Out1, Out2, Out3)"; portpinstr "Port Pin String"; blockid "Block ID"; inputporttype "Input Port Type"; inputportwidth "Input Port Width"; inputportlabel "Input Port Label"; outputporttype "Output Port Type"; outputportwidth "Output Port Width"; outputportlabel "Output port label"; compat "Compatibility (Reserved for future use)"; optionstring "String(s) to be passed to TLC"
      mask help:
      | The block define variables name for EEProm emulation on Flash memory.
      |
      | Note: maximum variable count limited to 48
      mask init:
      | stm32f0_eep_emulation_callback('init');
      mask Help: web(fullfile(waijungdocroot,'stm32f0_eep_emulation_storage.htm'), '-browser')
      mask StyleString: popup(Setup|Read|Write),popup(double|single|int8|uint8|int16|uint16|int32|uint32),edit,popup(<empty>),edit,edit,edit,edit,edit,edit,checkbox,edit,edit,edit,edit,edit,edit,edit,edit,edit,edit,edit,edit
      mask CallbackString: stm32f0_eep_emulation_callback('conf');||stm32f0_eep_emulation_callback('storagedefinename');||stm32f0_eep_emulation_callback('varname');|||stm32f0_eep_emulation_callback('eepfilename');||stm32f0_eep_emulation_callback('sampletime');|stm32f0_eep_emulation_callback('enablecustomportlabel');|stm32f0_eep_emulation_callback('conf');|stm32f0_eep_emulation_callback('conf');||stm32f0_eep_emulation_callback('blockid');||||||||
      mask Display: text(0.5, 0.5, '[EEP Setup]\nName: CAN_ID\nType: uint32','ver','middle','hor','center');
  Volatile Data Array : waijung_addon_module/Data Storage/Volatile Data Array  conf=Setup  specificaddress=off  storagename=READ_DATA  memoryaddress=hex2dec('64000000')  storagetype=uint8  datasize=256  varname=VolatileDataArray_READ_DATA  datatype=double  datacount=0  portpinstr=0  sampletime=inf  blockid=MemoryConfigurationVolatileDataArray  inputporttype=[]  inputportwidth=[]  inputportlabel={}  outputporttype=[]  outputportwidth=[]  outputportlabel={}  compat=0  optionstring="[\"off\",\"?\",\"READ_DATA\",\"uint8\",\"256\",\"VolatileDataArray_READ_DATA\",\"uint8_t\",\"Param1\"]"
  Volatile Data Array1 : waijung_addon_module/Data Storage/Volatile Data Array  conf=Setup  specificaddress=off  storagename=SLAVE_DEV_ID  memoryaddress=hex2dec('64000000')  storagetype=uint8  datasize=16  varname=VolatileDataArray_SLAVE_DEV_ID  datatype=double  datacount=0  portpinstr=0  sampletime=inf  blockid=MemoryConfigurationVolatileDataArray1  inputporttype=[]  inputportwidth=[]  inputportlabel={}  outputporttype=[]  outputportwidth=[]  outputportlabel={}  compat=0  optionstring="[\"off\",\"?\",\"SLAVE_DEV_ID\",\"uint8\",\"16\",\"VolatileDataArray_SLAVE_DEV_ID\",\"uint8_t\",\"Param1\"]"
  Volatile Data Array2 : waijung_addon_module/Data Storage/Volatile Data Array  conf=Setup  specificaddress=off  storagename=CONTROL  memoryaddress=hex2dec('64000000')  storagetype=uint8  datasize=256  varname=VolatileDataArray_CONTROL  datatype=double  datacount=0  portpinstr=0  sampletime=inf  blockid=MemoryConfigurationVolatileDataArray2  inputporttype=[]  inputportwidth=[]  inputportlabel={}  outputporttype=[]  outputportwidth=[]  outputportlabel={}  compat=0  optionstring="[\"off\",\"?\",\"CONTROL\",\"uint8\",\"256\",\"VolatileDataArray_CONTROL\",\"uint8_t\",\"Param1\"]"

== system stm32f0_ccp_sensor/Network/Interface Configuration ==
  CAN Setup : stm32f0_can_lib/CAN Setup  conf=Setup  canmodule=1  advance=off  bitrate_select=250000  sjw=1tq  bs1=15tq  bs2=8tq  timingconf=Prescaler  brp=8  bitrate=250000  tq=1.6667e-007  autoretransmission=Disable  remaptxpin=B9  remaprxpin=B8  sampletime=-1  sampletimestr=0.01  blockid=NetworkInterfaceConfigurationCANSetup  inputarray=[]  inputlabelarray={}  outputarray=[]  outputlabelarray={}  compat=0  confstr="[\"250000\",\"8\",\"B\",\"9\",\"B\",\"8\",\"1tq\",\"15tq\",\"8tq\",\"ENABLE\"]"  presc=8  txportstr=B  txpinstr=9  rxportstr=B  rxpinstr=8  lastmodule=1
  CAN_ID Configuration : Subsystem
  Soft I2C Master Setup : waijung_soft_i2c_lib/Soft I2C Master Setup  conf=Setup  targetname=stm32f0  module=1  transfer=Blocking  clk=250  timeout=25  sdapins='B7'  sclpins='B6'  writecount=1  readcount=1  waittime=0  forcestop=off  portpinstr=0  sampletime=-1  blockid=NetworkInterfaceConfigurationSoftI2CMasterSetup  inputporttype=[]  inputportwidth=[]  inputportlabel={}  outputporttype=[]  outputportwidth=[]  outputportlabel={}  compat=0  optionstring="[\"1\",\"250000\",\"3\",\"2\",\"1\",\"1\",\"25\",\"\",\"\",\"\",\"0\",\"1\",\"0\",\"0\",\"0\",\"0\",\"0\",\"0\",\"0\",\"\",\"1\",\"B\",\"7\",\"B\",\"6\"]"
  UART Setup : S-Function  FunctionName=stm32f0_uart  Parameters=conf,inputporttype,inputportwidth,outputporttype,outputportwidth,asciiheader,optionstring,headerstring,terminatorstring,asciidatatypestring,sampletime,blockid  EnableBusSupport=off  mask(stm32f0_uart){conf=Setup, uartmodule=1, baudrate=1000000, databits=8, parity=No, stopbit=1, remaptxpin=A9, remaprxpin=A10, flowcontrol=None, remapctspin=Not used, remaprtspin=Not used, advanceoptions=on, rxbuffersize=64, txbuffersize=64, transfer=Non-Blocking, packetmode=Binary, binheader='7E 7E', binterminator='03 03', porttype_double=1, porttype_single=1, porttype_int8=0, porttype_uint8=0, porttype_int16=0, porttype_uint16=1, porttype_int32=0, porttype_uint32=0, asciiformat='%1.2f', rx_asciiterminator=CR (0x0D - "\r"), tx_asciiterminator=CR (0x0D - "\r"), storagename=<empty>, varname=, asciiheader=, sampletime=-1, enablecustomportlabel=off, cinputportlabel=de, coutputportlabel=fff,ff,sdfsd, portpinstr=0, blockid=NetworkInterfaceConfigurationUARTSetup, inputporttype=[], inputportwidth=[], inputportlabel={}, outputporttype=[], outputportwidth=[], outputportlabel={}, compat=0, optionstring=["1", "1", "A", "9", "1", "A", "10", "0", "*", "*", "0", "*", "*", "1", "1", "", "", "1000000", "8", "No", "1", "None", "3", "2", "64", "64", "Binary", "Non-Blocking", ""], headerstring=[], terminatorstring=[], asciidatatypestring=[], lastmodule=1}
      mask prompts: conf "Configuration"; uartmodule "UART Module"; baudrate "Baud rate (bps)"; databits "Data bits"; stopbit "Stop bit"; remaptxpin "Tx pin"; remaprxpin "Rx pin"; flowcontrol "Hardware flow control"; remapctspin "HW Flow control, CTS Pin"; remaprtspin "HW Flow control, RTS Pin"; advanceoptions "Advance options"; rxbuffersize "Rx buffer size (bytes)"; txbuffersize "Tx buffer size (bytes)"; packetmode "Packet mode"; binheader "Binary header (example: '7E 7E')"; binterminator "Binary terminator (example: '03 03')"; porttype_double "Number of data port, type DOUBLE"; porttype_single "Number of data port, type SINGLE"; porttype_int8 "Number of data port, type INT8"; porttype_uint8 "Number of data port, type UINT8"; porttype_int16 "Number of data port, type INT16"; porttype_uint16 "Number of data port, type UINT16"; porttype_int32 "Number of data port, type INT32"; porttype_uint32 "Number of data port, type UINT32"; asciiformat "Ascii format"; rx_asciiterminator "End of packet"; tx_asciiterminator "End of packet"; storagename "Buffer"; varname "Var name"; asciiheader "Ascii header (printf format)"; sampletime "Sample time (sec)"; enablecustomportlabel "Enable custom port labels (Ex. In1, In2, In3)"; cinputportlabel "Custom input port labels (Ex. In1, In2, In3)"; coutputportlabel "Custom output port labels (Ex. Out1, Out2, Out3)"; portpinstr "Port Pin String"; blockid "Block ID"; inputporttype "Input Port Type"; inputportwidth "Input Port Width"; inputportlabel "Input Port Label"; outputporttype "Output Port Type"; outputportwidth "Output Port Width"; outputportlabel "Output port label"; compat "Compatibility (Reserved for future use)"; optionstring "String(s) to be passed to TLC"; lastmodule "Last module selected"
      mask help:
      | Default configuration for aMG USB Connect board:
      |  - UART module: 1
      |  - Tx pin: A9
      |  - Rx pin: A10
      |
      | Advance options
      |  - Rx buffer size (bytes): max packet length can be received via DMA.
      |  - Tx buffer size (bytes): max packet length can be transmit via DMA.
      mask init:
      | stm32f0_uart_callback('init');
      mask Help: web(fullfile(waijungdocroot,'stm32f0_uart_setup.htm'), '-browser')
      mask StyleString: popup(Setup|Tx|Rx),popup(1|2|3|4),edit,popup(8),popup(No|Odd|Even),popup(0.5|1|1.5|2),popup(Not used|A9|B6),popup(Not used|A10|B7),popup(None|RTS|CTS|RTS/CTS),popup(Not used|A11),popup(Not used|A12),checkbox,popup(16|32|64|128|256|512),popup(16|32|64|128|256|512),popup(Blocking|Non-Blocking),popup(Ascii|Binary|String Buffer),edit,edit,edit,edit,edit,edit,edit,edit,edit,edit,edit,popup(CR (0x0D - "\r")|LF (0x0A - "\n")|CRLF (0x0D 0x0A - "\r\n")),popup(CR (0x0D - "\r")|LF (0x0A - "\n")|CRLF (0x0D 0x0A - "\r\n")|None),popup(<empty>),edit,edit,edit,checkbox,edit,edit,edit,edit,edit,edit,edit,edit,edit,edit,edit,edit,edit,edit,edit,edit
      mask CallbackString: stm32f0_uart_callback('conf');|stm32f0_uart_callback('uartmodule');|||||||stm32f0_uart_callback('flowcontrol');|||stm32f0_uart_callback('advanceoptions');|||stm32f0_uart_callback('conf');|stm32f0_uart_callback('conf');|stm32f0_uart_callback('binheader');|stm32f0_uart_callback('binterminator');|||||||||stm32f0_uart_callback('asciiformat');|||stm32f0_uart_callback('storagename');|||stm32f0_uart_callback('sampletime');|stm32f0_uart_callback('enablecustomportlabel');|stm32f0_uart_callback('conf');|stm32f0_uart_callback('conf');||stm32f0_uart_callback('blockid');||||||||||||
      mask Display: text(0.5, 0.5, 'Module: USART1_Setup\nBaud (Bps): 1000000\nDMA Buffer: 64/64\nTx/Rx Pin: A9/A10','ver','middle','hor','center');

== system stm32f0_ccp_sensor/CAN Response/Reboot ==
  Enable : EnablePort
  System Reset : stm32f0_reset_lib/System Reset  conf=<empty>  sampletime=inf  sampletimestr=0.01  blockid=CANResponseRebootSystemReset  inputarray=[]  inputlabelarray={}  outputarray=[]  outputlabelarray={}  compat=0  confstr="[\"Param1\",\"Param1\"]"

== system stm32f0_ccp_sensor/CAN_ID/Subsystem ==
  Enable : EnablePort
  Constant : Constant  Value=0  OutDataTypeMode=uint8  OutDataType=fixdt(1, 16)  OutScaling=2^0  OutDataTypeStr=uint8
  EEP Emulation Read : S-Function  FunctionName=stm32f0_eep_emulation  Parameters=conf,inputporttype,inputportwidth,outputporttype,outputportwidth,eepfilename,eepinfo,varname,optionstring,sampletime,blockid  EnableBusSupport=off  mask(stm32f0_eep_emulation){conf=Read, datatype=single, storagedefinename='Data1,Data2', storagename=CAN_ID, varname='CAN_ID', initialvalue=[1.0 2.0], storageindex=0, eepfilename='stm32f0_ccp_sensor.eeprom', eepinfo='CAN_ID,7,0,-', debuginfo=off, sampletime=inf, enablecustomportlabel=off, cinputportlabel=0, coutputportlabel=, portpinstr=0, blockid=CAN_IDSubsystemEEPEmulationRead, inputporttype=[], inputportwidth=[], inputportlabel={}, outputporttype=[7], outputportwidth=[], outputportlabel={'CAN_ID'}, compat=0, optionstring=["CAN_ID","0","7","off","","","","","","","2","CAN_ID","7","0","dummy","0","0"]}
      mask prompts: conf "Configuration"; datatype "Storage type"; storagedefinename "Storage name"; storagename "Storage name"; varname "Var name (hidden)"; initialvalue "Initial value"; storageindex "Storage name index (hidden)"; eepfilename "EEP file name (hidden)"; eepinfo "EEP Information (hidden), [name, initialvalue, datatype]"; debuginfo "Debug information"; sampletime "Sample time (sec)"; enablecustomportlabel "Enable custom port labels (Ex. In1, In2, In3)"; cinputportlabel "Custom input port labels (Ex. In1, In2, In3)"; coutputportlabel "Custom output port labels (Ex. Out1, Out2, Out3)"; portpinstr "Port Pin String"; blockid "Block ID"; inputporttype "Input Port Type"; inputportwidth "Input Port Width"; inputportlabel "Input Port Label"; outputporttype "Output Port Type"; outputportwidth "Output Port Width"; outputportlabel "Output port label"; compat "Compatibility (Reserved for future use)"; optionstring "String(s) to be passed to TLC"
      mask help: Read a value from EEProm Emulation of the specified variable anme.
      mask init:
      | stm32f0_eep_emulation_callback('init');
      mask Help: web(fullfile(waijungdocroot,'stm32f0_eep_emulation_read.htm'), '-browser')
      mask StyleString: popup(Setup|Read|Write),popup(double|single|int8|uint8|int16|uint16|int32|uint32),edit,popup(CAN_ID),edit,edit,edit,edit,edit,checkbox,edit,checkbox,edit,edit,edit,edit,edit,edit,edit,edit,edit,edit,edit,edit
      mask CallbackString: stm32f0_eep_emulation_callback('conf');||stm32f0_eep_emulation_callback('storagedefinename');||stm32f0_eep_emulation_callback('varname');|||stm32f0_eep_emulation_callback('eepfilename');||stm32f0_eep_emulation_callback('debuginfo');|stm32f0_eep_emulation_callback('sampletime');|stm32f0_eep_emulation_callback('enablecustomportlabel');|stm32f0_eep_emulation_callback('conf');|stm32f0_eep_emulation_callback('conf');||stm32f0_eep_emulation_callback('blockid');||||||||
      mask Display: text(0.5, 0.5, '[EEP Read]\nName: CAN_ID\nTs (sec): 0.01','ver','middle','hor','center'); port_label('output', 1,'CAN_ID');
  FirstTime : Outport
  ID : Outport  Port=2  InitialOutput=0
  wires:
  EEP Emulation Read/1 -> ID/1
  Constant/1 -> FirstTime/1
